simulink model "Punto_2"  (R2024b)
settings: Solver=VariableStepAuto  StartTime=0.0  StopTime=10  RelTol=1e-3
settings Model: Creator=Andres Felipe  LastModifiedBy=Andres Felipe

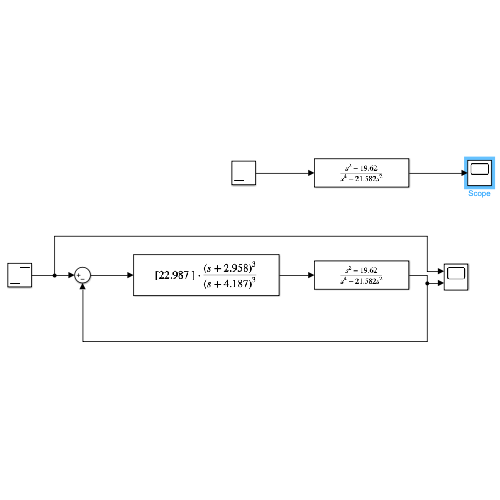
[thumbnail: Simulink's stored preview of the top-level diagram]
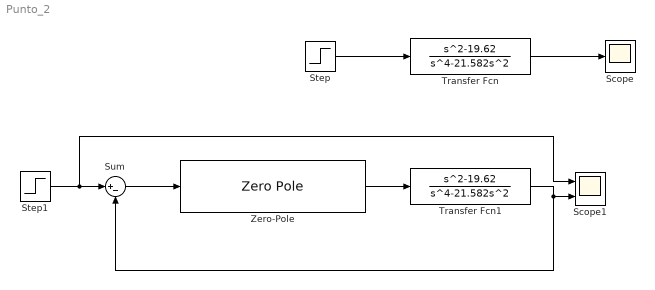
== system Punto_2 ==
  Scope : Scope
  Scope1 : Scope  NumInputPorts=2
  Step : Step  Time=0  SampleTime=0
  Step1 : Step  SampleTime=0
  Sum : Sum  Inputs=|+-
  Transfer Fcn : TransferFcn  Numerator=[1 0 -19.62]  Denominator=[1 0 -21.582 0 0]
  Transfer Fcn1 : TransferFcn  Numerator=[1 0 -19.62]  Denominator=[1 0 -21.582 0 0]
  Zero-Pole : ZeroPole  Zeros=[-2.958 -2.958 -2.958]  Poles=[-4.187 -4.187 -4.187]  Gain=[22.987]
  wires:
  Transfer Fcn/1 -> Scope/1
  Step/1 -> Transfer Fcn/1
  Zero-Pole/1 -> Transfer Fcn1/1
  Transfer Fcn1/1 -> Sum/2, Scope1/2
  Sum/1 -> Zero-Pole/1
  Step1/1 -> Scope1/1, Sum/1
